simulink model "chap02_03_62_mdl"  (R2013b)
settings: Solver=ode4  StartTime=0.0  StopTime=10  FixedStep=0.1  RelTol=1e-3
settings Model: Creator=Administrator  LastModifiedBy=sunzx.fnst

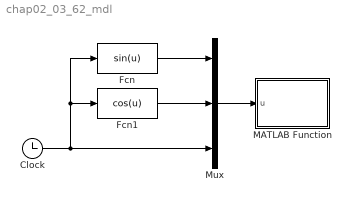
== system chap02_03_62_mdl ==
  Clock : Clock
  Fcn : Fcn  Expr=sin(u)
  Fcn1 : Fcn  Expr=cos(u)
  MATLAB Function : MATLAB Function  TreatAsAtomicUnit=on
  Mux : Mux  Inputs=3
  wires:
  Clock/1 -> Mux/3, Fcn/1, Fcn1/1
  Mux/1 -> MATLAB Function/1(u)
  Fcn/1 -> Mux/1
  Fcn1/1 -> Mux/2

== matlab function chap02_03_62_mdl/MATLAB Function ==
  data: u input
function scope_3d(u)
%#codegen
eml.extrinsic('plot3','scatter3','close','delete');
len = length(u);
persistent data
if isempty(data)
    data = zeros(3,100000);
end
persistent n   % count the input sample number
if isempty(n)
  n = 1;
else
  n = n + 1;
end
data(:,n) = u;
persistent h
if isempty(h)
    h = plot3(data(1,:),data(2,:),data(3,:),'o');
else
    delete(h);
    h = plot3(data(1,:),data(2,:),data(3,:),'o');
end
grid on;
